simulink model "pm_foc_models_digital"  (R2022b)
settings: Solver=VariableStepAuto  StartTime=0.0  StopTime=2  FixedStep=0.0001  RelTol=1e-3
values from neighbouring files (symbols this model uses):
  B = 0.0005    [pm_params.m]
  J = 0.0002    [pm_params.m]
  Lamda_f = 0.123    [pm_params.m]
  Ld = 0.0057    [pm_params.m]
  Lq = 0.0125    [pm_params.m]
  pole = 4    [pm_params.m]
  Rs = 1.2    [pm_params.m]
undefined symbols (not defined in the file or in its folder): sigbuilder_block
settings Model: Creator=jack  LastModifiedBy=jack

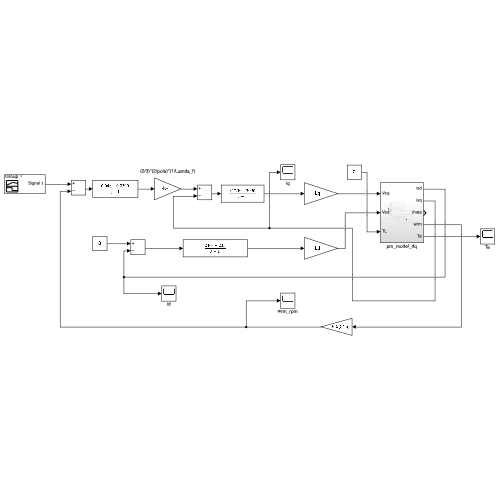
[thumbnail: Simulink's stored preview of the top-level diagram]
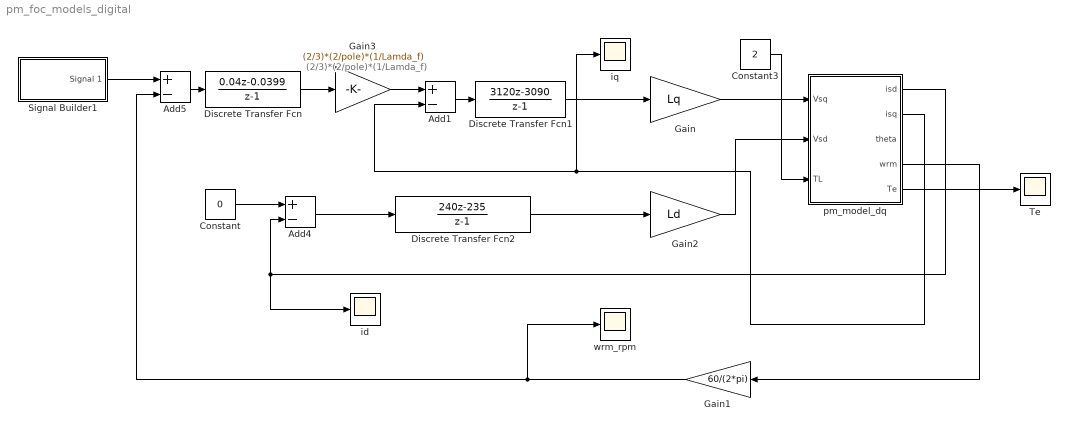
== system pm_foc_models_digital ==
  note: (2/3)*(2/pole)*(1/Lamda_f)
  Add1 : Sum  Inputs=+-
  Add4 : Sum  Inputs=+-
  Add5 : Sum  Inputs=+-
  Constant : Constant  Value=0
  Constant3 : Constant  Value=2
  Discrete Transfer Fcn : DiscreteTransferFcn  Numerator=[0.04 -0.0399]  Denominator=[1 -1]  SampleTime=0.001
  Discrete Transfer Fcn1 : DiscreteTransferFcn  Numerator=[3120 -3090]  Denominator=[1 -1]  SampleTime=0.0001
  Discrete Transfer Fcn2 : DiscreteTransferFcn  Numerator=[240 -235]  Denominator=[1 -1]  SampleTime=0.0001
  Gain : Gain  Gain=Lq
  Gain1 : Gain  Gain=60/(2*pi)
  Gain2 : Gain  Gain=Ld
  Gain3 : Gain  Gain=(2/3)*(2/pole)*(1/Lamda_f)
  Signal Builder1 : Subsystem  Tag=STV Subsys  LoadFcn=sigbuilder_block('load');  StartFcn=sigbuilder_block('start');  StopFcn=sigbuilder_block('stop');  ClipboardFcn=sigbuilder_block('clipboard');  mask(Sigbuilder block){tuvar=[0:10]}
      mask help: Simulink:masks:SigbuilderBlock_MD
      mask init:
      | if ~strcmp(get_param(bdroot(gcbh),'SimulationStatus'),'stopped') tuvar = sigbuilder_block('maskInit'); end
      settings: CopyFcn=sigbuilder_block('copy');  DeleteFcn=sigbuilder_block('delete');  ModelCloseFcn=sigbuilder_block('modelClose');  PreSaveFcn=sigbuilder_block('preSave');  PauseFcn=sigbuilder_block('pause');  ContinueFcn=sigbuilder_block('continue');  NameChangeFcn=sigbuilder_block('namechange');  OpenFcn=sigbuilder_block('open',[346 179 550 400 ]);  CloseFcn=sigbuilder_block('close');
      mask Display: plot(0, 0, 100, 100,[2, 2, 32, 32, 2], [68, 8, 8, 68, 68],[32, 2], [38, 38], [32, 19, 2],[53, 60, 44], [32, 17, 17, 2],[16, 16, 31, 31]);txt = getActiveGroup(gcbh);text(2, 100, txt,'verticalAlignment', 'top');
  Te : Scope
  id : Scope
  iq : Scope
  pm_model_dq : Subsystem
  wrm_rpm : Scope
  wires:
  Discrete Transfer Fcn/1 -> Gain3/1
  Add1/1 -> Discrete Transfer Fcn1/1
  Constant/1 -> Add4/1
  Add4/1 -> Discrete Transfer Fcn2/1
  Add5/1 -> Discrete Transfer Fcn/1
  Signal Builder1/1(Signal 1) -> Add5/1
  Gain1/1 -> wrm_rpm/1, Add5/2
  Gain/1 -> pm_model_dq/1(Vsq)
  pm_model_dq/2(isq) -> iq/1, Add1/2
  pm_model_dq/1(isd) -> Add4/2, id/1
  Gain2/1 -> pm_model_dq/2(Vsd)
  Constant3/1 -> pm_model_dq/3(TL)
  pm_model_dq/5(Te) -> Te/1
  pm_model_dq/4(wrm) -> Gain1/1
  Discrete Transfer Fcn2/1 -> Gain2/1
  Discrete Transfer Fcn1/1 -> Gain/1
  Gain3/1 -> Add1/1

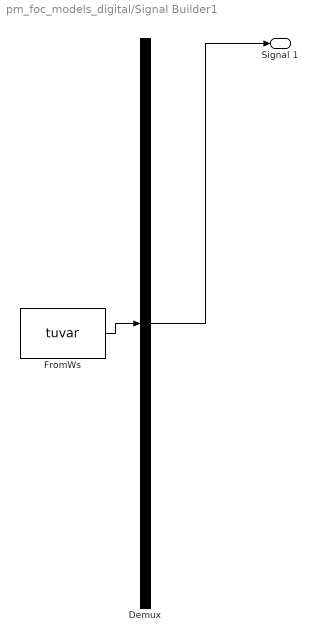
== system pm_foc_models_digital/Signal Builder1 ==
  Demux : Demux  Tag=STV Demux  Outputs=1
      settings: DisplayOption=none
  FromWs : FromWorkspace  Tag=STV FromWs  VariableName=tuvar
      SigBuilderData=|
      | common.afterFinalStr = 'Extrapolate'
      | common.sampleTime = 0
      | dataSet.timeRange = [0 10]
      | dataSet.name = 'Group 1'
      | sbobj.Groups.Name = 'Group 1'
      | sbobj.Groups.Signals.Name = 'Signal 1'
      | sbobj.Groups.Signals.XData = [0 1 4 6 10]
      | sbobj.Groups.Signals.YData = [0 1000 1000 1000 1000]
  Signal 1 : Outport  Tag=STV Outport
  wires:
  Demux/1 -> Signal 1/1
  FromWs/1 -> Demux/1

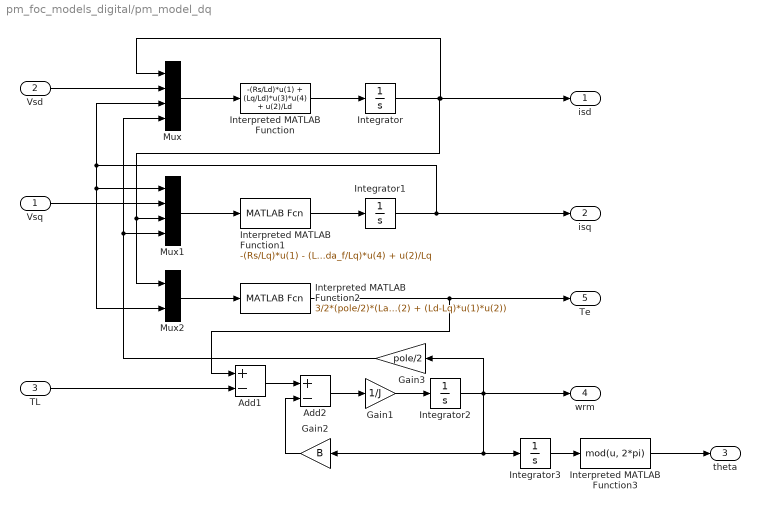
== system pm_foc_models_digital/pm_model_dq ==
  Vsq : Inport
  Vsd : Inport  Port=2
  TL : Inport  Port=3
  Add1 : Sum  Inputs=+-
  Add2 : Sum  Inputs=+-
  Gain1 : Gain  Gain=1/J
  Gain2 : Gain  Gain=B
  Gain3 : Gain  Gain=pole/2
  Integrator{,1..3} (4 alike) : Integrator
  Interpreted MATLAB Function : MATLABFcn  MATLABFcn=-(Rs/Ld)*u(1) + (Lq/Ld)*u(3)*u(4) + u(2)/Ld
  Interpreted MATLAB Function1 : MATLABFcn  MATLABFcn=-(Rs/Lq)*u(1) - (Ld/Lq)*u(3)*u(4) - (Lamda_f/Lq)*u(4) + u(2)/Lq
  Interpreted MATLAB Function2 : MATLABFcn  MATLABFcn=3/2*(pole/2)*(Lamda_f*u(2) + (Ld-Lq)*u(1)*u(2))
  Interpreted MATLAB Function3 : MATLABFcn  MATLABFcn=mod(u, 2*pi)
  Mux : Mux
  Mux1 : Mux
  Mux2 : Mux  Inputs=2
  isd : Outport
  isq : Outport  Port=2
  theta : Outport  Port=3
  wrm : Outport  Port=4
  Te : Outport  Port=5
  wires:
  Mux/1 -> Interpreted MATLAB Function/1
  Interpreted MATLAB Function1/1 -> Integrator1/1
  TL/1 -> Add1/2
  Vsd/1 -> Mux/2
  Integrator1/1 -> isq/1, Mux/3, Mux2/2, Mux1/1
  Interpreted MATLAB Function2/1 -> Te/1, Add1/1
  Gain3/1 -> Mux/4, Mux1/4
  Add2/1 -> Gain1/1
  Gain1/1 -> Integrator2/1
  Add1/1 -> Add2/1
  Mux2/1 -> Interpreted MATLAB Function2/1
  Interpreted MATLAB Function/1 -> Integrator/1
  Vsq/1 -> Mux1/2
  Integrator/1 -> Mux2/1, Mux1/3, isd/1, Mux/1
  Integrator2/1 -> wrm/1, Gain3/1, Integrator3/1, Gain2/1
  Interpreted MATLAB Function3/1 -> theta/1
  Mux1/1 -> Interpreted MATLAB Function1/1
  Gain2/1 -> Add2/2
  Integrator3/1 -> Interpreted MATLAB Function3/1
